simulink model "test_bus_test"  (R2020a)
settings: Solver=FixedStepDiscrete  StartTime=0.0  StopTime=2  FixedStep=Ts  RelTol=1e-3
model workspace (MAT data in the model file):
  p = Simulink.Parameter
  p.Value.ts = embedded.fi
  p.Value.ts.DataType = 'Fixed'
  p.Value.ts.Scaling = 'SlopeBias'
  p.Value.ts.Signed = 0
  p.Value.ts.WordLength = 32
  p.Value.ts.FixedExponent = -10
  p.Value.ts.SlopeAdjustmentFactor = 1.024
  p.Value.ts.Bias = 0
  p.Value.ts.DataTypeOverride = 'Inherit'
  p.Value.ts.intarray = 20
  p.Value.ts.noverflows = 0
  p.Value.ts.nunderflows = 0
  p.Value.ts.maxlog = -1.79769313486e+308
  p.Value.ts.minlog = 1.79769313486e+308
  p.Value.ts.RoundingMethod = 'Nearest'
  p.Value.ts.OverflowAction = 'Saturate'
  p.Value.ts.ProductMode = 'FullPrecision'
  p.Value.ts.SumMode = 'FullPrecision'
  p.Value.ts.ProductWordLength = 32
  p.Value.ts.SumWordLength = 32
  p.Value.ts.MaxProductWordLength = 65535
  p.Value.ts.MaxSumWordLength = 65535
  p.Value.ts.ProductFractionLength = 30
  p.Value.ts.ProductFixedExponent = -30
  p.Value.ts.ProductSlope = 9.31322574615e-10
  p.Value.ts.ProductSlopeAdjustmentFactor = 1
  p.Value.ts.ProductBias = 0
  p.Value.ts.SumFractionLength = 30
  p.Value.ts.SumFixedExponent = -30
  p.Value.ts.SumSlope = 9.31322574615e-10
  p.Value.ts.SumSlopeAdjustmentFactor = 1
  p.Value.ts.SumBias = 0
  p.Value.ts.CastBeforeSum = 1
  p.Value.ts.DDGMaxProductWordLength = 65535
  p.Value.ts.DDGMaxSumWordLength = 65535
  p.Value.ts.DDGProductFixedExponent = -30
  p.Value.ts.DDGProductFractionLength = 30
  p.Value.ts.DDGProductWordLength = 32
  p.Value.ts.DDGSumFixedExponent = -30
  p.Value.ts.DDGSumFractionLength = 30
  p.Value.ts.DDGSumWordLength = 32
  p.Value.ts.DDGCastBeforeSum = 1
  p.Value.ts.DDGProductBias = 0
  p.Value.ts.DDGProductSlopeAdjustmentFactor = 1
  p.Value.ts.DDGSumBias = 0
  p.Value.ts.DDGSumSlopeAdjustmentFactor = 1
  p.Value.ts.DDGProductSlope = 9.31322574615e-10
  p.Value.ts.DDGSumSlope = 9.31322574615e-10
  p.Value.ts.Logging = 0
  p.Value.ts.fimathislocal = 0
  p.Value.Para1 = embedded.fi
  p.Value.Para1.DataType = 'Fixed'
  p.Value.Para1.Scaling = 'SlopeBias'
  p.Value.Para1.Signed = 0
  p.Value.Para1.WordLength = 32
  p.Value.Para1.FixedExponent = 0
  p.Value.Para1.SlopeAdjustmentFactor = 1
  p.Value.Para1.Bias = 0
  p.Value.Para1.DataTypeOverride = 'Inherit'
  p.Value.Para1.intarray = 2
  p.Value.Para1.noverflows = 0
  p.Value.Para1.nunderflows = 0
  p.Value.Para1.maxlog = -1.79769313486e+308
  p.Value.Para1.minlog = 1.79769313486e+308
  p.Value.Para1.RoundingMethod = 'Nearest'
  p.Value.Para1.OverflowAction = 'Saturate'
  p.Value.Para1.ProductMode = 'FullPrecision'
  p.Value.Para1.SumMode = 'FullPrecision'
  p.Value.Para1.ProductWordLength = 32
  p.Value.Para1.SumWordLength = 32
  p.Value.Para1.MaxProductWordLength = 65535
  p.Value.Para1.MaxSumWordLength = 65535
  p.Value.Para1.ProductFractionLength = 30
  p.Value.Para1.ProductFixedExponent = -30
  p.Value.Para1.ProductSlope = 9.31322574615e-10
  p.Value.Para1.ProductSlopeAdjustmentFactor = 1
  p.Value.Para1.ProductBias = 0
  p.Value.Para1.SumFractionLength = 30
  p.Value.Para1.SumFixedExponent = -30
  p.Value.Para1.SumSlope = 9.31322574615e-10
  p.Value.Para1.SumSlopeAdjustmentFactor = 1
  p.Value.Para1.SumBias = 0
  p.Value.Para1.CastBeforeSum = 1
  p.Value.Para1.DDGMaxProductWordLength = 65535
  p.Value.Para1.DDGMaxSumWordLength = 65535
  p.Value.Para1.DDGProductFixedExponent = -30
  p.Value.Para1.DDGProductFractionLength = 30
  p.Value.Para1.DDGProductWordLength = 32
  p.Value.Para1.DDGSumFixedExponent = -30
  p.Value.Para1.DDGSumFractionLength = 30
  p.Value.Para1.DDGSumWordLength = 32
  p.Value.Para1.DDGCastBeforeSum = 1
  p.Value.Para1.DDGProductBias = 0
  p.Value.Para1.DDGProductSlopeAdjustmentFactor = 1
  p.Value.Para1.DDGSumBias = 0
  p.Value.Para1.DDGSumSlopeAdjustmentFactor = 1
  p.Value.Para1.DDGProductSlope = 9.31322574615e-10
  p.Value.Para1.DDGSumSlope = 9.31322574615e-10
  p.Value.Para1.Logging = 0
  p.Value.Para1.fimathislocal = 0
  p.Value.Para2 = embedded.fi
  p.Value.Para2.DataType = 'Fixed'
  p.Value.Para2.Scaling = 'SlopeBias'
  p.Value.Para2.Signed = 0
  p.Value.Para2.WordLength = 16
  p.Value.Para2.FixedExponent = 0
  p.Value.Para2.SlopeAdjustmentFactor = 1
  p.Value.Para2.Bias = 0
  p.Value.Para2.DataTypeOverride = 'Inherit'
  p.Value.Para2.intarray = 4
  p.Value.Para2.noverflows = 0
  p.Value.Para2.nunderflows = 0
  p.Value.Para2.maxlog = -1.79769313486e+308
  p.Value.Para2.minlog = 1.79769313486e+308
  p.Value.Para2.RoundingMethod = 'Nearest'
  p.Value.Para2.OverflowAction = 'Saturate'
  p.Value.Para2.ProductMode = 'FullPrecision'
  p.Value.Para2.SumMode = 'FullPrecision'
  p.Value.Para2.ProductWordLength = 32
  p.Value.Para2.SumWordLength = 32
  p.Value.Para2.MaxProductWordLength = 65535
  p.Value.Para2.MaxSumWordLength = 65535
  p.Value.Para2.ProductFractionLength = 30
  p.Value.Para2.ProductFixedExponent = -30
  p.Value.Para2.ProductSlope = 9.31322574615e-10
  p.Value.Para2.ProductSlopeAdjustmentFactor = 1
  p.Value.Para2.ProductBias = 0
  p.Value.Para2.SumFractionLength = 30
  p.Value.Para2.SumFixedExponent = -30
  p.Value.Para2.SumSlope = 9.31322574615e-10
  p.Value.Para2.SumSlopeAdjustmentFactor = 1
  p.Value.Para2.SumBias = 0
  p.Value.Para2.CastBeforeSum = 1
  p.Value.Para2.DDGMaxProductWordLength = 65535
  p.Value.Para2.DDGMaxSumWordLength = 65535
  p.Value.Para2.DDGProductFixedExponent = -30
  p.Value.Para2.DDGProductFractionLength = 30
  p.Value.Para2.DDGProductWordLength = 32
  p.Value.Para2.DDGSumFixedExponent = -30
  p.Value.Para2.DDGSumFractionLength = 30
  p.Value.Para2.DDGSumWordLength = 32
  p.Value.Para2.DDGCastBeforeSum = 1
  p.Value.Para2.DDGProductBias = 0
  p.Value.Para2.DDGProductSlopeAdjustmentFactor = 1
  p.Value.Para2.DDGSumBias = 0
  p.Value.Para2.DDGSumSlopeAdjustmentFactor = 1
  p.Value.Para2.DDGProductSlope = 9.31322574615e-10
  p.Value.Para2.DDGSumSlope = 9.31322574615e-10
  p.Value.Para2.Logging = 0
  p.Value.Para2.fimathislocal = 0
  p.Value.TimeDelay = embedded.fi
  p.Value.TimeDelay.DataType = 'Fixed'
  p.Value.TimeDelay.Scaling = 'SlopeBias'
  p.Value.TimeDelay.Signed = 0
  p.Value.TimeDelay.WordLength = 32
  p.Value.TimeDelay.FixedExponent = 0
  p.Value.TimeDelay.SlopeAdjustmentFactor = 1
  p.Value.TimeDelay.Bias = 0
  p.Value.TimeDelay.DataTypeOverride = 'Inherit'
  p.Value.TimeDelay.intarray = 0
  p.Value.TimeDelay.noverflows = 0
  p.Value.TimeDelay.nunderflows = 0
  p.Value.TimeDelay.maxlog = -1.79769313486e+308
  p.Value.TimeDelay.minlog = 1.79769313486e+308
  p.Value.TimeDelay.RoundingMethod = 'Nearest'
  p.Value.TimeDelay.OverflowAction = 'Saturate'
  p.Value.TimeDelay.ProductMode = 'FullPrecision'
  p.Value.TimeDelay.SumMode = 'FullPrecision'
  p.Value.TimeDelay.ProductWordLength = 32
  p.Value.TimeDelay.SumWordLength = 32
  p.Value.TimeDelay.MaxProductWordLength = 65535
  p.Value.TimeDelay.MaxSumWordLength = 65535
  p.Value.TimeDelay.ProductFractionLength = 30
  p.Value.TimeDelay.ProductFixedExponent = -30
  p.Value.TimeDelay.ProductSlope = 9.31322574615e-10
  p.Value.TimeDelay.ProductSlopeAdjustmentFactor = 1
  p.Value.TimeDelay.ProductBias = 0
  p.Value.TimeDelay.SumFractionLength = 30
  p.Value.TimeDelay.SumFixedExponent = -30
  p.Value.TimeDelay.SumSlope = 9.31322574615e-10
  p.Value.TimeDelay.SumSlopeAdjustmentFactor = 1
  p.Value.TimeDelay.SumBias = 0
  p.Value.TimeDelay.CastBeforeSum = 1
  p.Value.TimeDelay.DDGMaxProductWordLength = 65535
  p.Value.TimeDelay.DDGMaxSumWordLength = 65535
  p.Value.TimeDelay.DDGProductFixedExponent = -30
  p.Value.TimeDelay.DDGProductFractionLength = 30
  p.Value.TimeDelay.DDGProductWordLength = 32
  p.Value.TimeDelay.DDGSumFixedExponent = -30
  p.Value.TimeDelay.DDGSumFractionLength = 30
  p.Value.TimeDelay.DDGSumWordLength = 32
  p.Value.TimeDelay.DDGCastBeforeSum = 1
  p.Value.TimeDelay.DDGProductBias = 0
  p.Value.TimeDelay.DDGProductSlopeAdjustmentFactor = 1
  p.Value.TimeDelay.DDGSumBias = 0
  p.Value.TimeDelay.DDGSumSlopeAdjustmentFactor = 1
  p.Value.TimeDelay.DDGProductSlope = 9.31322574615e-10
  p.Value.TimeDelay.DDGSumSlope = 9.31322574615e-10
  p.Value.TimeDelay.Logging = 0
  p.Value.TimeDelay.fimathislocal = 0
  p.Value.num = [0 1]
  p.Value.den = [0 1]
  p.Description = 'Parameter structure for model: bus_test'
  p.DataType = 'Bus: bus_test_Para_t'
  p.Dimensions = [1 1]
settings Model: ParameterArgumentNames=p  OrderedModelArguments=off  Creator=C3038028  LastModifiedBy=w.schwamm
settings DataIOCC: SaveFormat=Array  SaveOutput=off  SignalLogging=off  DSMLogging=off  SaveTime=off  ReturnWorkspaceOutputs=off  SignalLoggingName=sigsOut
settings OptimizationCC: DefaultParameterBehavior=Inlined  InlineInvariantSignals=on  EnhancedBackFolding=on  ExpressionDepthLimit=2147483647  StateBitsets=on  DataBitsets=on  ZeroExternalMemoryAtStartup=off  NoFixptDivByZeroProtection=on  EfficientFloat2IntCast=on  EfficientMapNaN2IntZero=off  LifeSpan=1  BufferReusableBoundary=off  EfficientTunableParamExpr=on
settings DebuggingCC: MergeDetectMultiDrivingBlocksExec=none  CheckExecutionContextPreStartOutputMsg=on  CheckExecutionContextRuntimeOutputMsg=on  IntegerOverflowMsg=none  FcnCallInpInsideContextMsg=warning  AllowSymbolicDim=off  StateNameClashWarn=warning  StrictBusMsg=ErrorOnBusTreatedAsVector  SymbolicDimsDataTypeCodeGenerationDiagnostic=none  SFUnexpectedBacktrackingDiag=warning  SFNoUnconditionalDefaultTransitionDiag=warning  SFExecutionAtInitializationDiag=none  IntegerSaturationMsg=none  ArithmeticOperatorsInVariantConditions=warning
settings HardwareCC: TargetHWDeviceType=Generic->32-bit Embedded Processor
settings ModelReferenceCC: UpdateModelReferenceTargets=IfOutOfDate  PropagateSignalLabelsOutOfModel=off
settings SFSimCC: SimUseLocalCustomCode=off  MATLABDynamicMemAlloc=off
settings RTWCC: Description=Embedded Coder (host-based shared library target)  SystemTargetFile=ert_shrlib.tlc  TLCOptions=-p0 -aWarnNonSaturatedBlocks=0  TemplateMakefile=ert_default_tmf  RTWVerbose=off  RTWUseLocalCustomCode=off
settings CodeAppCC: ForceParamTrailComments=on  IgnoreCustomStorageClasses=off  IgnoreTestpoints=on  CustomSymbolStrType=$N$R$M  StateflowObjectComments=on  InternalIdentifier=Classic
settings STFCustomTargetCC: TargetFcnLib=ansi_tfl_tmw.mat  GenerateSampleERTMain=on  ParMdlRefBuildCompliant=on  CompOptLevelCompliant=on  CombineOutputUpdateFcns=on  SuppressErrorStatus=on  ERTCustomFileBanners=on  SupportAbsoluteTime=off  MultiInstanceERTCode=on  CodeInterfacePackaging=Reusable function  SupportNonFinite=off  SupportComplex=off  SupportContinuousTime=off  SupportNonInlinedSFcns=off  RemoveResetFunc=on  MATLABClassNameForMDSCustomization=Simulink.SoftwareTarget.ERTCustomization  ModelStepFunctionPrototypeControlCompliant=on  CPPClassGenCompliant=on  UseToolchainInfoCompliant=on  SystemTargetFile=ert_shrlib.tlc
settings ERTTargetCC: TargetFcnLib=ansi_tfl_tmw.mat  MultiwordLength=2048  GenerateSampleERTMain=on  ConcurrentExecutionCompliant=off  SuppressErrorStatus=on  SupportAbsoluteTime=off  MultiInstanceERTCode=on  CodeInterfacePackaging=Reusable function  SupportNonFinite=off  SupportComplex=off  ExtModeMexFile=noextcomm  InlinedParameterPlacement=NonHierarchical  RootIOFormat=Structure reference  ERTCustomFileTemplate=example_file_process.tlc  ERTFilePackagingFormat=CompactWithDataFile  ConvertIfToSwitch=off  SuppressUnreachableDefaultCases=off
settings ConfigComp: CovMetricSettings=d  CovHtmlReporting=on  CovSaveCumulativeToWorkspaceVar=on  CovSaveSingleToWorkspaceVar=on  CovExternalEMLEnable=off

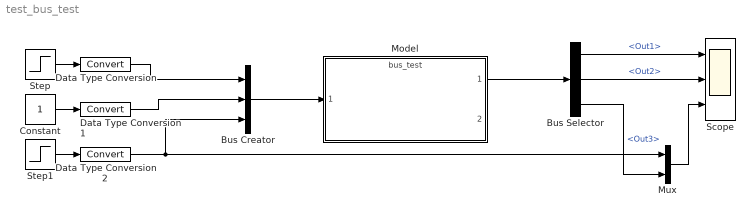
== system test_bus_test ==
  Bus Creator : BusCreator  Inputs=3  OutDataTypeStr=Bus: bus_test_In_t  NonVirtualBus=on
      settings: InheritFromInputs=off
  Bus Selector : BusSelector  OutputSignals=Out1,Out2,Out3
  Constant : Constant
  Data Type Conversion : DataTypeConversion
  Data Type Conversion1 : DataTypeConversion
  Data Type Conversion2 : DataTypeConversion
  Model : ModelReference  ModelNameDialog=bus_test.mdl  ParameterArgumentNames=p  ParameterArgumentValues=bus_test_Para  UsingDefaultArgumentValue=0  SimulationMode=Normal  ModelReferenceVersion=1.59
  Mux : Mux  Inputs=2
  Scope : Scope  NumInputPorts=3
  Step : Step  SampleTime=0
  Step1 : Step  SampleTime=0
  wires:
  Bus Creator/1 -> Model/1
  Step/1 -> Data Type Conversion/1
  Constant/1 -> Data Type Conversion1/1
  Step1/1 -> Data Type Conversion2/1
  Data Type Conversion/1 -> Bus Creator/1
  Data Type Conversion1/1 -> Bus Creator/2
  Data Type Conversion2/1 -> Bus Creator/3, Mux/1
  Model/1 -> Bus Selector/1
  Bus Selector/1 -> Scope/1  "<Out1>"
  Bus Selector/2 -> Scope/2  "<Out2>"
  Bus Selector/3 -> Mux/2  "<Out3>"
  Mux/1 -> Scope/3
